simulink model "COMPARISON_f"  (R2015b)
settings: Solver=ode45  StartTime=0.0  StopTime=2  RelTol=1e-3
settings Model: Creator=japerez  LastModifiedBy=d.alazard
settings DataIOCC: SaveFormat=Array
settings DebuggingCC: SolverPrmCheckMsg=warning
settings HardwareCC: ProdBitPerPointer=32  ProdLargestAtomicFloat=None  ProdIntDivRoundTo=Undefined  ProdEndianess=Unspecified  ProdWordSize=32  ProdHWDeviceType=32-bit Generic
settings GRTTargetCC: GeneratePreprocessorConditionals=Disable all
settings ConfigComp: CovModelRefEnable=Off  CovSFcnEnable=off

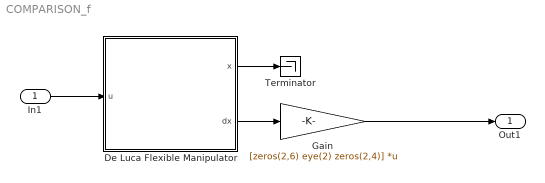
== system COMPARISON_f ==
  In1 : Inport
  De Luca Flexible Manipulator : Subsystem
  Gain : Gain  Gain=[zeros(2,6) eye(2) zeros(2,4)]  Multiplication=Matrix(K*u) (u vector)
  Terminator : Terminator
  Out1 : Outport
  wires:
  In1/1 -> De Luca Flexible Manipulator/1(u)
  De Luca Flexible Manipulator/1(x) -> Terminator/1
  De Luca Flexible Manipulator/2(dx) -> Gain/1
  Gain/1 -> Out1/1

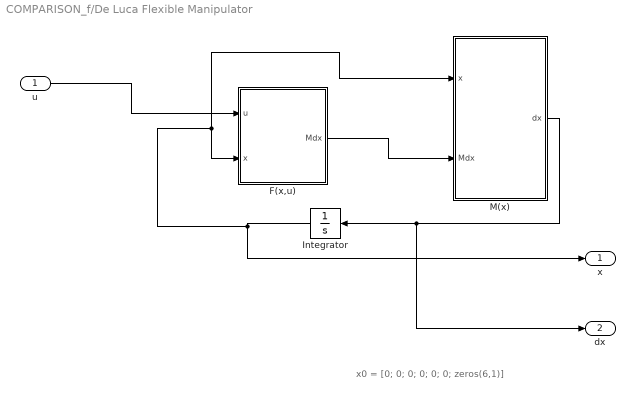
== system COMPARISON_f/De Luca Flexible Manipulator ==
  note: x0 = [0; 0; 0; 0; 0; 0; zeros(6,1)]
  u : Inport  PortDimensions=2
  F(x,u) : MATLAB Function  TreatAsAtomicUnit=on
  Integrator : Integrator  InitialCondition=[0; 0; 0; 0; 0; 0; zeros(6,1)]
  M(x) : MATLAB Function  TreatAsAtomicUnit=on
  x : Outport
  dx : Outport  Port=2
  wires:
  u/1 -> F(x,u)/1(u)
  Integrator/1 -> M(x)/1(x), F(x,u)/2(x), x/1
  M(x)/1(dx) -> dx/1, Integrator/1
  F(x,u)/1(Mdx) -> M(x)/2(Mdx)

== matlab function COMPARISON_f/De Luca Flexible Manipulator/F(x,u) ==
  data: u input; Mdx output; x input
function Mdx = F(u,x)
% FOR SIMULINK ONLY
%  Evaluates the right side of the differential equations of the two-link 
% flexible manipulator proposed by De Luca and Siciliano:"Closed-Form Dynamic Model Planar Multilink
% Lightweight Robots", IEEE Transactions of systems Vol 21, N°4, 1991
%
% F(t,x,u) = F(q,dq,u) = -h(q,dq) -Kq + Qu
%
% Inputs: 
%
%       u: input vector 
%       x: state vector, x = (q,dq)' with q = (theta1,theta2,delta11,delta12
%          ,delta21,delta22)'
%
% Outputs: dx (state vector derivate)
%
% Auxiliar functions: u = U(time) (actuators at the joints)
%
% Last revision:
% J. Alvaro Perez 23rd May 2016
%
% % Verification examples: Watch the graphics of the original paper
%--------------------------------------------------------------------------

%% NOT CLEAN:initialize constants manually and not by argument

rho1 = 0.2; % Kg/m
rho2 = 0.2; % Kg/m

l1 = 0.5; % m
l2 = 0.5; % m
d2 = 0.25; % m

m1 = 0.1; % Kg
m2 = 0.1; % Kg
mh2 = 1.0; % Kg
mp = 0.1; % Kg

Jo1 = 0.0083; % Kgm2
Jo2 = 0.0083; % Kgm2
Jh1 = 0.1; % Kgm2
Jh2 = 0.1; % Kgm2
Jp = 0.0005; % Kgm2

EI1 = 1; % Nm2;
EI2 = 1; % Nm2; 

% Parameters coming for the AMM for the nominal configuration:
phi11e = 0.186;
phi12e = 0.215;
phi_t_11e = 0.657;
phi_t_12e = -0.560;
phi21e = 0.883;
phi22e = -0.069;
phi_t_21e = 2.641;
phi_t_22e = -10.853;

v11 = 0.007;
v12 = 0.013;
v21 = 0.033;
v22 = 0.054;

w11 = 0.002;
w12 = 0.004;
w21 = 0.012;
w22 = 0.016;

f11 = 0.48; % Hz
f12 = 1.80; % Hz
f21 = 2.18; % Hz
f22 = 15.91; % Hz

% K matrix computation for the nominal configuration
K = diag([0,0, (2*pi*f11)^2*m1, (2*pi*f12)^2*m1, (2*pi*f21)^2*m2, (2*pi*f22)^2*m2]);

% Q matrix computation for the nominal configuration
Q = [eye(2); zeros(4,2)];

% t coefficients

t11 = phi11e - l1*phi_t_11e;
t12 = phi12e - l1*phi_t_12e;
t21 = v21 + mp*phi21e;
t22 = v22 + mp*phi22e;
t31 = phi_t_11e;
t32 = phi_t_12e;

% h coefficients: First Round!
%

h101 = -2*(m2*d2 + mp*l2)*l1;
h102 = 2*(m2*d2 + mp*l2)*(phi11e - l1*phi_t_11e);
h103 = 2*(m2*d2 + mp*l2)*(phi12e - l1*phi_t_12e);
h104 = -2*(v21 + mp*phi21e)*l1;
h105 = -2*(v22 + mp*phi22e)*l1;
h106 = -(m2*d2 + mp*l2)*l1;
h107 = -(m2*d2 + mp*l2)*l1*phi_t_11e;
h108 = -2*(m2*d2 + mp*l2)*l1*phi_t_12e;
h109 = -2*(v21 + mp*phi21e)*l1;
h110 = -2*(v22 + mp*phi22e)*l1;
h111 = -2*(v21 + mp*phi21e)*l1*phi_t_11e;
h112 = -2*(v22 + mp*phi22e)*l1*phi_t_11e;
h113 = -2*(v21 + mp*phi21e)*l1*phi_t_12e;
h114 = -2*(v22 + mp*phi22e)*l1*phi_t_12e;
h115 = 2*(m2*d2 + mp*l2);
h116 = m2*d2 + mp*l2;
h117 = -(v21 + mp*phi21e);
h118 = -(v22 + mp*phi22e);
h119 = -2*l1;
h120 = -l1;
h121 = -(phi11e + l1*phi_t_11e);
h122 = -(phi12e + l1*phi_t_12e);
h123 = -(m2*d2 + mp*l2)*(phi11e*phi_t_12e - phi12e*phi_t_11e);
h124 = -(m2*d2 + mp*l2)*(phi12e*phi_t_11e - phi11e*phi_t_12e);

% h coefficients: Second Round!
%

h201 = (m2*d2 + mp*l2)*l1;
h202 = 2*(m2*d2 + mp*l2)*phi11e;
h203 = 2*(m2*d2 + mp*l2)*phi12e;
h204 = -(m2*d2 + mp*l2);
h205 = -(v21 + mp*phi21e);
h206 = -(v22 + mp*phi22e);
h207 = l1;
h208 = phi11e + l1*phi_t_11e;
h209 = phi12e + l1*phi_t_12e;
h210 = (m2*d2 + mp*l2)*(phi11e*phi_t_12e - phi12e*phi_t_11e);
h211 = (m2*d2 + mp*l2)*(phi12e*phi_t_11e - phi11e*phi_t_12e);
h212 = phi11e*phi_t_11e;
h213 = phi11e*phi_t_12e + phi12e*phi_t_11e;
h214 = (v21 + mp*phi21e)*phi11e;
h215 = (v22 + mp*phi22e)*phi11e;
h216 = phi12e*phi_t_12e;
h217 = (v21 + mp*phi21e)*phi12e;
h218 = (v22 + mp*phi22e)*phi12e;

% h coefficients: Third Round!
%

h301 = -(m2*d2 + mp*l2)*(phi11e - l1*phi_t_11e);
h302 = -2*(m2*d2 + mp*l2)*phi11e;
h303 = 2*(m2*d2 + mp*l2)*(phi12e*phi_t_11e - phi11e*phi_t_12e);
h304 = -2*(v21 + mp*phi21e)*phi11e;
h305 = -2*(v22 + mp*phi22e)*phi11e;
h306 = -(m2*d2 + mp*l2)*phi11e;
h307 = -2*(m2*d2 + mp*l2)*phi11e*phi_t_11e;
h308 = -2*(m2*d2 + mp*l2)*phi11e*phi_t_12e;
h309 = -2*(v21 + mp*phi21e)*phi11e;
h310 = -2*(v22 + mp*phi22e)*phi11e;
h311 = -2*(v21 + mp*phi21e)*phi11e*phi_t_11e;
h312 = -2*(v22 + mp*phi22e)*phi11e*phi_t_11e;
h313 = -2*(v21 + mp*phi21e)*phi11e*phi_t_12e;
h314 = -2*(v22 + mp*phi22e)*phi11e*phi_t_12e;
h315 = -(phi11e + l1*phi_t_11e);
h316 = -phi11e;
h317 = -2*phi11e*phi_t_11e;
h318 = -(phi11e*phi_t_12e + phi12e*phi_t_11e);
h319 = -(m2*d2 + mp*l2)*phi11e;
h320 = -(v21 + mp*phi21e)*phi11e;
h321 = -(v22 + mp*phi22e)*phi11e;
h322 = -(m2*d2 +mp*l2)*(phi11e*phi_t_12e - phi12e*phi_t_11e);

% h coefficients: Fourth Round!
%

h401 = -(m2*d2 + mp*l2)*(phi12e - l1*phi_t_12e);
h402 = -2*(m2*d2 + mp*l2)*phi12e;
h403 = 2*(m2*d2 + mp*l2)*(phi11e*phi_t_12e - phi12e*phi_t_11e);
h404 = -2*(v21 + mp*phi21e)*phi12e;
h405 = -2*(v22 + mp*phi22e)*phi12e;
h406 = -(m2*d2 + mp*l2)*phi12e;
h407 = -2*(m2*d2 + mp*l2)*phi12e*phi_t_11e;
h408 = -2*(m2*d2 + mp*l2)*phi12e*phi_t_12e;
h409 = -2*(v21 + mp*phi21e)*phi12e;
h410 = -2*(v22 + mp*phi22e)*phi12e;
h411 = -2*(v21 + mp*phi21e)*phi12e*phi_t_11e;
h412 = -2*(v22 + mp*phi22e)*phi12e*phi_t_12e;
h413 = -2*(v21 + mp*phi21e)*phi12e*phi_t_11e;
h414 = -2*(v22 + mp*phi22e)*phi12e*phi_t_12e;
h415 = -(phi12e + l1*phi_t_12e);
h416 = -phi12e;
h417 = -(phi11e*phi_t_12e + phi12e*phi_t_11e);
h418 = -2*phi12e*phi_t_12e;
h419 = -(m2*d2 + mp*l2)*phi12e;
h420 = -(v21 + mp*phi21e)*phi12e;
h421 = -(v22 + mp*phi22e)*phi12e;
h422 = -(m2*d2 + mp*l2)*(phi12e*phi_t_11e - phi11e*phi_t_12e);


% h coefficients: Fifth Round!
%

h501 = (v21 + mp*phi21e)*l1;
h502 = 2*(v21 + mp*phi21e)*phi11e;
h503 = 2*(v21 + mp*phi21e)*phi12e;
h504 = v21 + mp*phi21e;
h505 = -(v21 + mp*phi21e)*phi11e;
h506 = -(v21 + mp*phi21e)*phi12e;

% h coefficients: Sixth Round!
%

h601 = (v22 + mp*phi22e)*l1;
h602 = 2*(v22 + mp*phi22e)*phi11e;
h603 = 2*(v22 + mp*phi22e)*phi12e;
h604 = v22 + mp*phi22e;
h605 = -(v22 + mp*phi22e)*phi11e;
h606 = -(v22 + mp*phi22e)*phi12e;



%% State variables definition x  = (q,dq) = (theta1,theta2,delta11,delta12
%  ,delta21,delta22,dtheta1, dtheta2,ddelta11,ddelta12,ddelta21,ddelta22)'



D11 = x(3); % delta11
D12 = x(4); % delta12
D21 = x(5); % delta21
D22 = x(6); % delta22

dt1 = x(7); % dtheta1
dt2 = x(8); % dtheta2
dD11 = x(9); % ddelta11
dD12 = x(10); % ddelta12
dD21 = x(11); % ddelta21
dD22 = x(12); % ddelta22

c2 = cos(x(2)); % cos(theta2)
s2 = sin(x(2)); % sin(theta2)
t1 = t11*D11 + t12*D12; % t1 = t11*delta11 + t12*delta12
t2 = t21*D21 + t22*D22; % t2 = t21*delta21 + t22*delta22
t3 = t31*D11 + t32*D12; % t3 = t31*delta11 + t32*delta12


% Computing h(q,dq);

h1 = ((h101*dt2 + h102*dD11 + h103*dD12 + h104*dD21 + h105*dD22)*dt1 +...
     (h106*dt2 + h107*dD11 + h108*dD12 + h109*dD21 + h110*dD22)*dt2 +...
     (h111*dD21 + h112*dD22)*dD11 + (h113*dD21 + h114*dD22)*dD12)*s2 + ...
     ((h115*dt1 + h116*dt2 + h117*dD21 +h118*dD22)*t1 +...
     (h119*dt1 + h120*dt2 + h121*dD11 +h122*dD12)*t2 +...
     h123*D12*dD11 + h124*D11*dD12)*dt2*c2;

h2 = (h201*dt1 + h202*dD11 + h203*dD12)*dt1*s2 + ...
     (((h204*dt1 + h205*dD21 + h206*dD22)*t1 +...
     (h207*dt1 + h208*dD11 + h209*dD12)*t2 + ...
      h210*D12*dD11 + h211*D11*dD12)*dt1 + ...
      ((h212*dD11 + h213*dD12)*t2 + (h214*dD21 + h215*dD22)*t3)*dD11 + ...
      (h216*dD12*t2 + (h217*dD21 + h218*dD22)*t3)*dD12)*c2;

h3 = ((h301*dt1 + h302*dt2 + h303*dD12 + h304*dD21 + h305*dD22)*dt1 + ...
      (h306*dt2 + h307*dD11 + h308*dD12 + h309*dD21 + h310*dD22)*dt2 + ...
       (h311*dD21 + h312*dD22)*dD11 + (h313*dD21 + h314*dD22)*dD12)*s2 + ...
       ((h315*dt1 + h316*dt2 + h317*dD11 + h318*dD12)*t2 + ...
       (h319*dt2 + h320*dD21 + h321*dD22)*t3 + h322*D12*dt1)*dt2*c2;

h4 = ((h401*dt1 + h402*dt2 + h403*dD11 + h404*dD21 + h405*dD22)*dt1 + ...
      (h406*dt2 + h407*dD11 + h408*dD12 + h409*dD21 + h410*dD22)*dt2 + ...
      (h411*dD21 + h412*dD22)*dD11 + (h413*dD21 + h414*dD22)*dD12)*s2 +...
      ((h415*dt1 + h416*dt2 + h417*dD11 + h418*dD12)*t2 + ...
       (h419*dt2 + h420*dD21 + h421*dD22)*t3 + h422*D11*dt1)*dt2*c2;
   
h5 = (h501*dt1 + h502*dD11 + h503*dD12)*dt1*s2 + ...
     (h504*t1*dt1 + (h505*dD11 + h506*dD12)*t3)*dt2*c2;

h6 = (h601*dt1 + h602*dD11 + h603*dD12)*dt1*s2 + ...
     (h604*t1*dt1 +(h605*dD11 + h606*dD12)*t3)*dt2*c2;

% Right hand of the M(t,y)y' = f(t,y) equation
H  = [h1; h2; h3; h4; h5; h6];
KX = K*x(1:6);
QU = Q*u;
Bddq = -H - KX + QU;

% Right hand of the dq/dt = dq/dt
dq = x(7:12);

% Final result
Mdx = [dq ;Bddq];


end
%#codegen

== matlab function COMPARISON_f/De Luca Flexible Manipulator/M(x) ==
  data: dx output; x input; Mdx input
function dx = MASS(x, Mdx)
% FOR SIMULINK ONLY
% Mass Matrix computation (B) of the two-link flexible manipulator proposed
% by De Luca and Siciliano:"Closed-Form Dynamic Model Planar Multilink
% Lightweight Robots", IEEE Transactions of systems Vol 21, N°4, 1991
%
% Inputs: 
%
%       t: time vector (Useless. For this case, B = B(q))
%       x: state vector, x = (q,dq)' with q = (theta1,theta2,delta11,delta12
%          ,delta21,delta22)'
%
% Outputs: Mass matrix B(q)
%
% Last revision:
% J. Alvaro Perez 23rd May 2016
%
% % Verification examples: Watch the graphics of the original paper
%--------------------------------------------------------------------------

%% NOT CLEAN:initialize constants manually and not by argument

rho1 = 0.2; % Kg/m
rho2 = 0.2; % Kg/m

l1 = 0.5; % m
l2 = 0.5; % m
d2 = 0.25; % m

m1 = 0.1; % Kg
m2 = 0.1; % Kg
mh2 = 1.0; % Kg
mp = 0.1; % Kg

Jo1 = 0.0083; % Kgm2
Jo2 = 0.0083; % Kgm2
Jh1 = 0.1; % Kgm2
Jh2 = 0.1; % Kgm2
Jp = 0.0005; % Kgm2

EI1 = 1; % Nm2;
EI2 = 1; % Nm2; 

% Parameters coming for the AMM for the nominal configuration:
phi11e = 0.186;
phi12e = 0.215;
phi_t_11e = 0.657;
phi_t_12e = -0.560;
phi21e = 0.883;
phi22e = -0.069;
phi_t_21e = 2.641;
phi_t_22e = -10.853;

v11 = 0.007;
v12 = 0.013;
v21 = 0.033;
v22 = 0.054;

w11 = 0.002;
w12 = 0.004;
w21 = 0.012;
w22 = 0.016;

f11 = 0.48; % Hz
f12 = 1.80; % Hz
f21 = 2.18; % Hz
f22 = 15.91; % Hz

% K matrix computation for the nominal configuration
K = diag([0,0, (2*pi*f11)^2*m1, (2*pi*f12)^2*m1, (2*pi*f21)^2*m2, (2*pi*f22)^2*m2]);

% Q matrix computation for the nominal configuration
Q = [eye(2); zeros(4,2)];

% b coefficients: First Round! 
%
b111 = Jh1 + Jo1 + Jh2 + mh2*l1^2 + Jo2 + m2*l1^2 + Jp + mp*(l1^2+l2^2);
b112 = 2*(m2*d2 + mp*l2)*l1;
b113 = 2*(m2*d2 + mp*l2);
b114 = -2*l1;
b121 = Jh2 + Jo2 + Jp + mp*l2^2;
b122 = (m2*d2 + mp*l2)*l1;
b123 = m2*d2 + mp*l2;
b124 = -l1;
b131 = w11 + (Jh2 + Jo2 + Jp + mp*l2^2)*phi_t_11e + (mh2 + m2 + mp)*l1*phi11e;
b132 = (m2*d2 + mp*l2)*(phi11e + l1*phi_t_11e);
b133 = -(phi11e + l1*phi_t_11e);
b134 = -(m2*d2 + mp*l2)*(phi11e*phi_t_12e - phi12e*phi_t_11e);
b141 = w12 + (Jh2 + Jo2 + Jp + mp*l2^2)*phi_t_12e + (mh2 + m2 + mp)*l1*phi12e;
b142 = (m2*d2 + mp*l2)*(phi12e + l1*phi_t_12e);
b143 = -(phi12e + l1*phi_t_12e);
b144 = -(m2*d2 + mp*l2)*(phi12e*phi_t_11e - phi11e*phi_t_12e);
b151 = w21 + Jp*phi_t_21e + mp*l2*phi21e;
b152 = (v21 + mp*phi21e)*l1;
b153 = v21 + mp*phi21e;
b161 = w22 + Jp*phi_t_22e + mp*l2*phi22e;
b162 = (v22 + mp*phi22e)*l1;
b163 = v22 + mp*phi22e;

% b coefficients: Second Round! 
%
b221 = Jh2 + Jo2 + Jp + mp*l2^2;
b231 = (Jh2 + Jo2 + Jp + mp*l2^2)*phi_t_11e;
b232 = (m2*d2 + mp*l2)*phi11e;
b233 = -phi11e;
b234 = -(m2*d2 + mp*l2)*phi11e;
b241 = (Jh2 + Jo2 + Jp + mp*l2^2)*phi_t_12e;
b242 = (m2*d2 + mp*l2)*phi12e;
b243 = -phi12e;
b244 = -(m2*d2 + mp*l2)*phi12e;
b251 = w21 + Jp*phi_t_21e + mp*l2*phi21e;
b261 = w22 + Jp*phi_t_22e + mp*l2*phi22e;

% b coefficients: Third Round! 
%

b331 = m1;
b332 = 2*(m2*d2 + mp*l2)*phi11e*phi_t_11e;
b333 = -2*phi11e*phi_t_11e;
b341 = 0;
b342 = (m2*d2 + mp*l2)*(phi11e*phi_t_12e + phi12e*phi_t_11e);
b343 = -(phi11e*phi_t_12e + phi12e*phi_t_11e);
b351 = (w21 + Jp*phi_t_21e + mp*l2*phi21e)*phi_t_11e;
b352 = (v21 + mp*phi21e)*phi11e;
b353 = -(v21 + mp*phi21e)*phi11e;
b361 = (w22 + Jp*phi_t_22e + mp*l2*phi22e)*phi_t_11e;
b362 = (v22 + mp*phi22e)*phi11e;
b363 = -(v22 + mp*phi22e)*phi11e;

% b coefficients: Fourth Round!
%

b441 = m1;
b442 = 2*(m2*d2 + mp*l2)*phi12e*phi_t_12e;
b443 = -2*phi12e*phi_t_12e;
b451 = (w21 + Jp*phi_t_21e + mp*l2*phi21e)*phi_t_12e;
b452 = (v21 + mp*phi21e)*phi12e;
b453 = -(v21 + mp*phi21e)*phi12e;
b461 = (w22 + Jp*phi_t_22e + mp*l2*phi22e)*phi_t_12e;
b462 = (v22 + mp*phi22e)*phi12e;
b463 = -(v22 + mp*phi22e)*phi12e;

b551 = m2;
b561 = 0;
b661 = m2;

% t coefficients

t11 = phi11e - l1*phi_t_11e;
t12 = phi12e - l1*phi_t_12e;
t21 = v21 + mp*phi21e;
t22 = v22 + mp*phi22e;
t31 = phi_t_11e;
t32 = phi_t_12e;

%% Real function
% Define useful variables:
c2 = cos(x(2)); % cos(theta2)
s2 = sin(x(2)); % sin(theta2)
t1 = t11*x(3) + t12*x(4); % t1 = t11*delta11 + t12*delta12
t2 = t21*x(5) + t22*x(6); % t2 = t21*delta21 + t22*delta22
t3 = t31*x(3) + t32*x(4); % t3 = t31*delta11 + t32*delta12

% Mass Matrix terms
B11 = b111 + b112*c2 + (b113*t1 + b114*t2)*s2;
B12 = b121 + b122*c2 + (b123*t1 + b124*t2)*s2;
B13 = b131 + b132*c2 + (b133*t2 + b134*x(4))*s2;
B14 = b141 + b142*c2 + (b143*t2 + b144*x(3))*s2;
B15 = b151 + b152*c2 + b153*t1*s2;
B16 = b161 + b162*c2 + b163*t1*s2;

B22 = b221;
B23 = b231 + b232*c2 + (b233*t2 + b234*t3)*s2;
B24 = b241 + b242*c2 + (b243*t2 + b244*t3)*s2;
B25 = b251;
B26 = b261;

B33 = b331 + b332*c2 + b333*t2*s2;
B34 = b341 + b342*c2 + b343*t2*s2;
B35 = b351 + b352*c2 + b353*t3*s2;
B36 = b361 + b362*c2 + b363*t3*s2;

B44 = b441 + b442*c2 + b443*t2*s2;
B45 = b451 + b452*c2 + b453*t3*s2;
B46 = b461 + b462*c2 + b463*t3*s2;

B55 = b551;
B56 = b561;

B66 = b661;

B = [B11 B12 B13 B14 B15 B16;
     B12 B22 B23 B24 B25 B26;
     B13 B23 B33 B34 B35 B36;
     B14 B24 B34 B44 B45 B46;
     B15 B25 B35 B45 B55 B56;
     B16 B26 B36 B46 B56 B66];

% Mass Matrix assembly (second order system) : 
M = [eye(6) zeros(6); zeros(6) B];

% Since M*dx/dt = F(x,t)
% The derivate of states is therefore
dx = inv(M)*Mdx;
end
